simulink model "MPCii_convertidorSEPIC"  (R2015a)
settings: Solver=ode45  StartTime=0.0  StopTime=0.1  RelTol=1e-3
values from neighbouring files (symbols this model uses):
  Ts = 1/(50e3)    (= 2e-05)    [MPCii.m]
undefined symbols (not defined in the file or in its folder): A, Ao, B, Bo, C, Co, Do
settings Model: Creator=estudiante  LastModifiedBy=berme_000

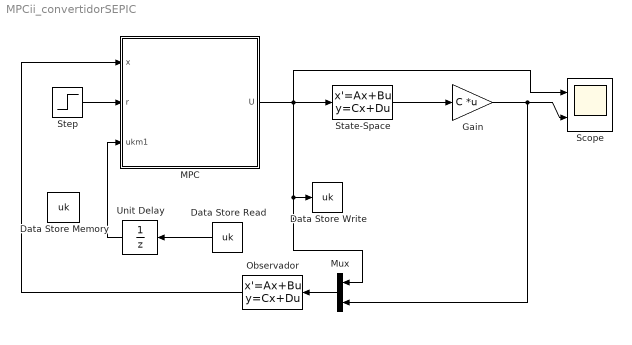
== system MPCii_convertidorSEPIC ==
  Data Store Memory : DataStoreMemory  DataStoreName=uk  ReadBeforeWriteMsg=warning  WriteAfterWriteMsg=warning  WriteAfterReadMsg=warning
  Data Store Read : DataStoreRead  DataStoreName=uk
  Data Store Write : DataStoreWrite  DataStoreName=uk
  Gain : Gain  Gain=C  Multiplication=Matrix(K*u)
  MPC : Subsystem
  Mux : Mux  Inputs=2
  Observador : StateSpace  A=Ao  B=Bo  C=Co  D=Do  X0=0
  Scope : Scope  NumInputPorts=2
      settings: YMin=0.348047~25.0025  YMax=0.348047~25.0025  SaveName=mpc_ml_ouput
  State-Space : StateSpace  A=A  B=B  C=eye(4)  D=zeros(4,1)  X0=0
  Step : Step  Time=0.05  Before=20  After=25  SampleTime=0
  Unit Delay : UnitDelay  SampleTime=-1
  wires:
  Step/1 -> MPC/2(r)
  Unit Delay/1 -> MPC/3(ukm1)
  Data Store Read/1 -> Unit Delay/1
  State-Space/1 -> Gain/1
  MPC/1(U) -> State-Space/1, Scope/1, Mux/1, Data Store Write/1
  Gain/1 -> Mux/2, Scope/2
  Observador/1 -> MPC/1(x)
  Mux/1 -> Observador/1

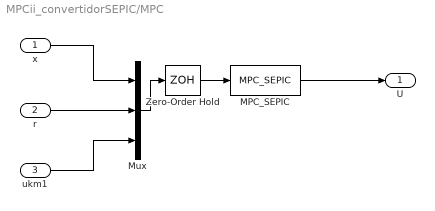
== system MPCii_convertidorSEPIC/MPC ==
  x : Inport  PortDimensions=4
  r : Inport  Port=2
  ukm1 : Inport  Port=3
  MPC_SEPIC : MATLABFcn  MATLABFcn=MPC_SEPIC
  Mux : Mux  Inputs=3
  Zero-Order Hold : ZeroOrderHold  SampleTime=Ts
  U : Outport
  wires:
  x/1 -> Mux/1
  r/1 -> Mux/2
  Mux/1 -> Zero-Order Hold/1
  Zero-Order Hold/1 -> MPC_SEPIC/1
  MPC_SEPIC/1 -> U/1
  ukm1/1 -> Mux/3
